simulink model "nuclearReactor"  (R2014b)
settings: Solver=ode1  StartTime=0.0  StopTime=100  FixedStep=0.0001  MaxStep=0.0001  RelTol=1e-3
(part 2 of 4)

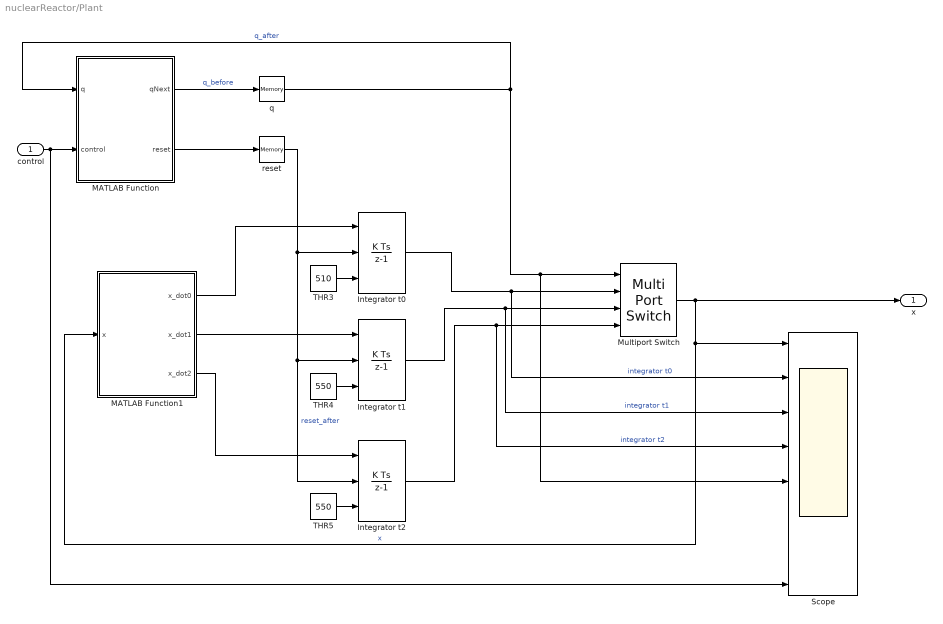
== system nuclearReactor/Plant ==
  control : Inport
  Integrator t0 : DiscreteIntegrator  ExternalReset=either  InitialConditionSource=external  InitialCondition=510  InitialConditionSetting=State (most efficient)  SampleTime=-1
  Integrator t1 : DiscreteIntegrator  ExternalReset=either  InitialConditionSource=external  InitialCondition=510  InitialConditionSetting=State (most efficient)  SampleTime=-1
  Integrator t2 : DiscreteIntegrator  ExternalReset=either  InitialConditionSource=external  InitialCondition=510  InitialConditionSetting=State (most efficient)  SampleTime=-1
  MATLAB Function : MATLAB Function  Priority=1  TreatAsAtomicUnit=on
  MATLAB Function1 : MATLAB Function  Priority=1  TreatAsAtomicUnit=on
  Multiport Switch : MultiPortSwitch  DataPortOrder=Zero-based contiguous
  Scope : Scope  NumInputPorts=8
      settings: TickLabels=on  ShowLegends=on  YMin=0~0~0~10~1~1~0~-1  YMax=40~20~20~30~3~3~1~1
  THR3 : Constant  Value=510
  THR4 : Constant  Value=550
  THR5 : Constant  Value=550
  q : Memory  LinearizeMemory=on
  reset : Memory  LinearizeMemory=on
  x : Outport
  wires:
  Multiport Switch/1 -> Scope/1, MATLAB Function1/1(x), x/1  "x"
  MATLAB Function1/1(x_dot0) -> Integrator t0/1
  THR3/1 -> Integrator t0/3
  THR4/1 -> Integrator t1/3
  THR5/1 -> Integrator t2/3
  Integrator t0/1 -> Scope/2, Multiport Switch/2  "integrator t0"
  Integrator t1/1 -> Scope/3, Multiport Switch/3  "integrator t1"
  Integrator t2/1 -> Scope/4, Multiport Switch/4  "integrator t2"
  MATLAB Function1/2(x_dot1) -> Integrator t1/1
  MATLAB Function1/3(x_dot2) -> Integrator t2/1
  MATLAB Function/1(qNext) -> q/1  "q_before"
  q/1 -> MATLAB Function/1(q), Scope/5, Multiport Switch/1  "q_after"
  control/1 -> Scope/8, MATLAB Function/2(control)
  MATLAB Function/2(reset) -> reset/1
  reset/1 -> Integrator t0/2, Integrator t1/2, Integrator t2/2  "reset_after"

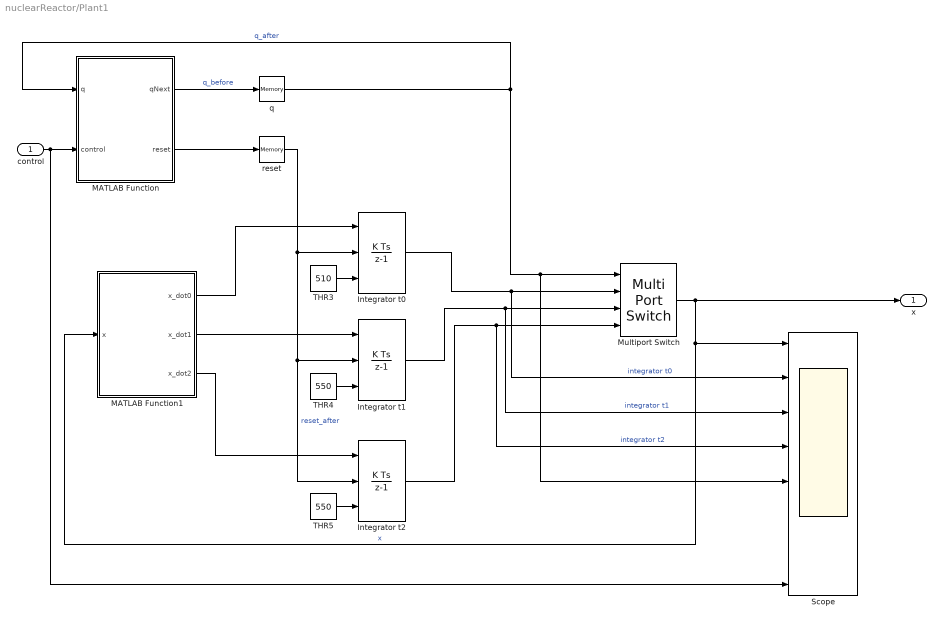
== system nuclearReactor/Plant1 ==
  control : Inport
  Integrator t0 : DiscreteIntegrator  ExternalReset=either  InitialConditionSource=external  InitialCondition=510  InitialConditionSetting=State (most efficient)  SampleTime=-1
  Integrator t1 : DiscreteIntegrator  ExternalReset=either  InitialConditionSource=external  InitialCondition=510  InitialConditionSetting=State (most efficient)  SampleTime=-1
  Integrator t2 : DiscreteIntegrator  ExternalReset=either  InitialConditionSource=external  InitialCondition=510  InitialConditionSetting=State (most efficient)  SampleTime=-1
  MATLAB Function : MATLAB Function  Priority=1  TreatAsAtomicUnit=on
  MATLAB Function1 : MATLAB Function  Priority=1  TreatAsAtomicUnit=on
  Multiport Switch : MultiPortSwitch  DataPortOrder=Zero-based contiguous
  Scope : Scope  NumInputPorts=8
      settings: TickLabels=on  ShowLegends=on  YMin=0~0~0~10~1~1~0~-1  YMax=40~20~20~30~3~3~1~1
  THR3 : Constant  Value=510
  THR4 : Constant  Value=550
  THR5 : Constant  Value=550
  q : Memory  LinearizeMemory=on
  reset : Memory  LinearizeMemory=on
  x : Outport
  wires:
  Multiport Switch/1 -> Scope/1, MATLAB Function1/1(x), x/1  "x"
  MATLAB Function1/1(x_dot0) -> Integrator t0/1
  THR3/1 -> Integrator t0/3
  THR4/1 -> Integrator t1/3
  THR5/1 -> Integrator t2/3
  Integrator t0/1 -> Scope/2, Multiport Switch/2  "integrator t0"
  Integrator t1/1 -> Scope/3, Multiport Switch/3  "integrator t1"
  Integrator t2/1 -> Scope/4, Multiport Switch/4  "integrator t2"
  MATLAB Function1/2(x_dot1) -> Integrator t1/1
  MATLAB Function1/3(x_dot2) -> Integrator t2/1
  MATLAB Function/1(qNext) -> q/1  "q_before"
  q/1 -> MATLAB Function/1(q), Scope/5, Multiport Switch/1  "q_after"
  control/1 -> Scope/8, MATLAB Function/2(control)
  MATLAB Function/2(reset) -> reset/1
  reset/1 -> Integrator t0/2, Integrator t1/2, Integrator t2/2  "reset_after"

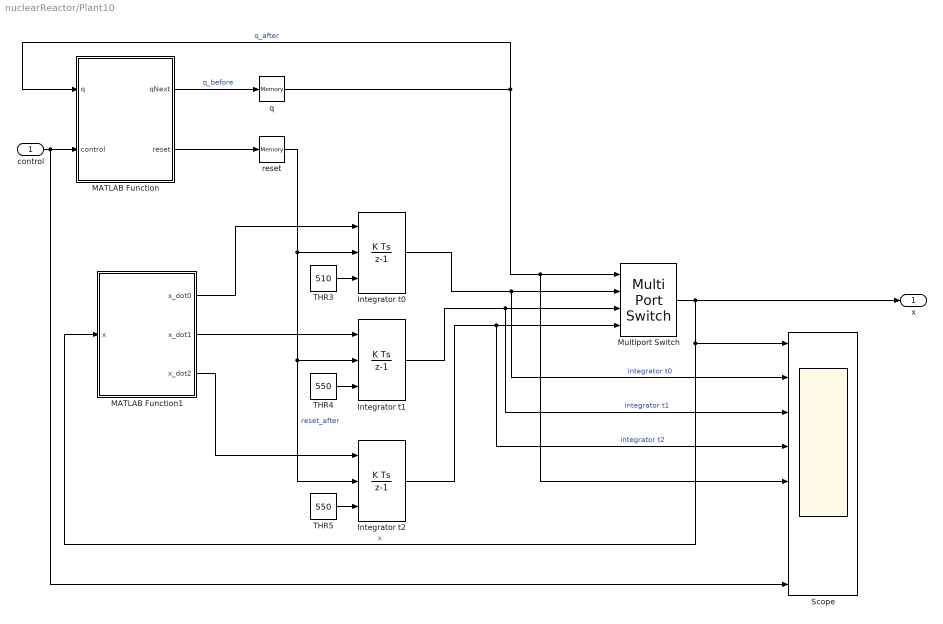
== system nuclearReactor/Plant10 ==
  control : Inport
  Integrator t0 : DiscreteIntegrator  ExternalReset=either  InitialConditionSource=external  InitialCondition=510  InitialConditionSetting=State (most efficient)  SampleTime=-1
  Integrator t1 : DiscreteIntegrator  ExternalReset=either  InitialConditionSource=external  InitialCondition=510  InitialConditionSetting=State (most efficient)  SampleTime=-1
  Integrator t2 : DiscreteIntegrator  ExternalReset=either  InitialConditionSource=external  InitialCondition=510  InitialConditionSetting=State (most efficient)  SampleTime=-1
  MATLAB Function : MATLAB Function  Priority=1  TreatAsAtomicUnit=on
  MATLAB Function1 : MATLAB Function  Priority=1  TreatAsAtomicUnit=on
  Multiport Switch : MultiPortSwitch  DataPortOrder=Zero-based contiguous
  Scope : Scope  NumInputPorts=8
      settings: TickLabels=on  ShowLegends=on  YMin=0~0~0~10~1~1~0~-1  YMax=40~20~20~30~3~3~1~1
  THR3 : Constant  Value=510
  THR4 : Constant  Value=550
  THR5 : Constant  Value=550
  q : Memory  LinearizeMemory=on
  reset : Memory  LinearizeMemory=on
  x : Outport
  wires:
  Multiport Switch/1 -> Scope/1, MATLAB Function1/1(x), x/1  "x"
  MATLAB Function1/1(x_dot0) -> Integrator t0/1
  THR3/1 -> Integrator t0/3
  THR4/1 -> Integrator t1/3
  THR5/1 -> Integrator t2/3
  Integrator t0/1 -> Scope/2, Multiport Switch/2  "integrator t0"
  Integrator t1/1 -> Scope/3, Multiport Switch/3  "integrator t1"
  Integrator t2/1 -> Scope/4, Multiport Switch/4  "integrator t2"
  MATLAB Function1/2(x_dot1) -> Integrator t1/1
  MATLAB Function1/3(x_dot2) -> Integrator t2/1
  MATLAB Function/1(qNext) -> q/1  "q_before"
  q/1 -> MATLAB Function/1(q), Scope/5, Multiport Switch/1  "q_after"
  control/1 -> Scope/8, MATLAB Function/2(control)
  MATLAB Function/2(reset) -> reset/1
  reset/1 -> Integrator t0/2, Integrator t1/2, Integrator t2/2  "reset_after"

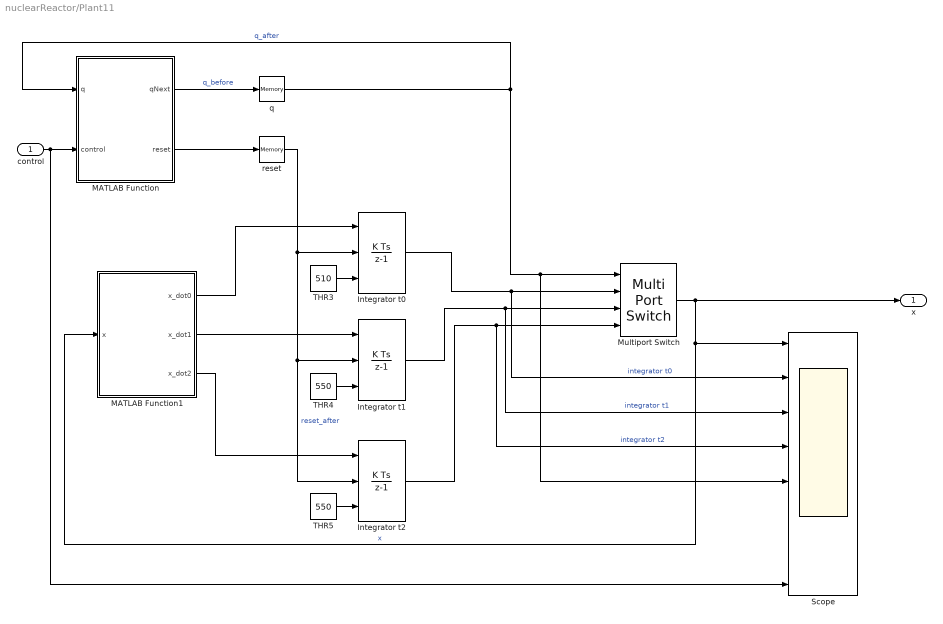
== system nuclearReactor/Plant11 ==
  control : Inport
  Integrator t0 : DiscreteIntegrator  ExternalReset=either  InitialConditionSource=external  InitialCondition=510  InitialConditionSetting=State (most efficient)  SampleTime=-1
  Integrator t1 : DiscreteIntegrator  ExternalReset=either  InitialConditionSource=external  InitialCondition=510  InitialConditionSetting=State (most efficient)  SampleTime=-1
  Integrator t2 : DiscreteIntegrator  ExternalReset=either  InitialConditionSource=external  InitialCondition=510  InitialConditionSetting=State (most efficient)  SampleTime=-1
  MATLAB Function : MATLAB Function  Priority=1  TreatAsAtomicUnit=on
  MATLAB Function1 : MATLAB Function  Priority=1  TreatAsAtomicUnit=on
  Multiport Switch : MultiPortSwitch  DataPortOrder=Zero-based contiguous
  Scope : Scope  NumInputPorts=8
      settings: TickLabels=on  ShowLegends=on  YMin=0~0~0~10~1~1~0~-1  YMax=40~20~20~30~3~3~1~1
  THR3 : Constant  Value=510
  THR4 : Constant  Value=550
  THR5 : Constant  Value=550
  q : Memory  LinearizeMemory=on
  reset : Memory  LinearizeMemory=on
  x : Outport
  wires:
  Multiport Switch/1 -> Scope/1, MATLAB Function1/1(x), x/1  "x"
  MATLAB Function1/1(x_dot0) -> Integrator t0/1
  THR3/1 -> Integrator t0/3
  THR4/1 -> Integrator t1/3
  THR5/1 -> Integrator t2/3
  Integrator t0/1 -> Scope/2, Multiport Switch/2  "integrator t0"
  Integrator t1/1 -> Scope/3, Multiport Switch/3  "integrator t1"
  Integrator t2/1 -> Scope/4, Multiport Switch/4  "integrator t2"
  MATLAB Function1/2(x_dot1) -> Integrator t1/1
  MATLAB Function1/3(x_dot2) -> Integrator t2/1
  MATLAB Function/1(qNext) -> q/1  "q_before"
  q/1 -> MATLAB Function/1(q), Scope/5, Multiport Switch/1  "q_after"
  control/1 -> Scope/8, MATLAB Function/2(control)
  MATLAB Function/2(reset) -> reset/1
  reset/1 -> Integrator t0/2, Integrator t1/2, Integrator t2/2  "reset_after"

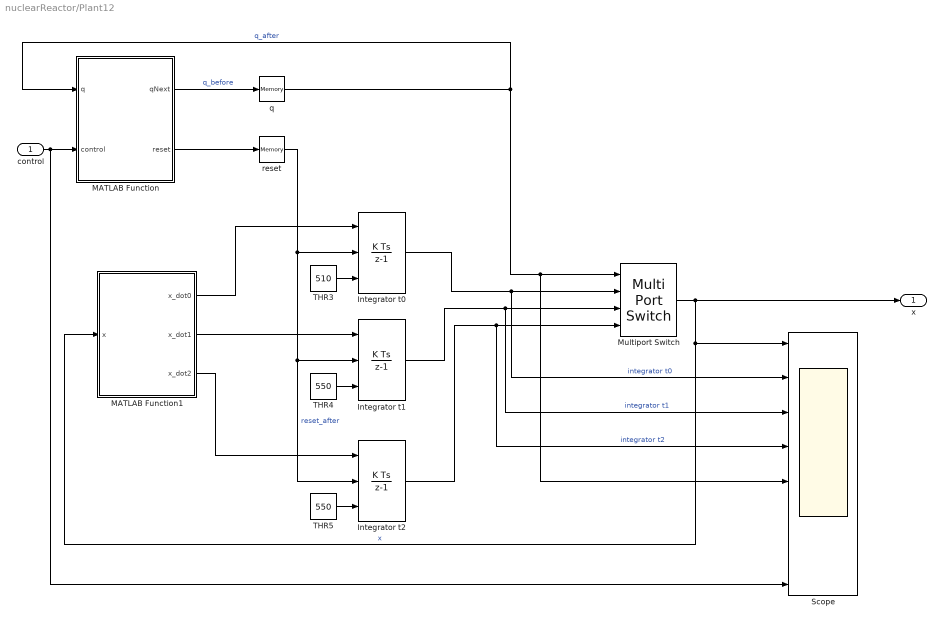
== system nuclearReactor/Plant12 ==
  control : Inport
  Integrator t0 : DiscreteIntegrator  ExternalReset=either  InitialConditionSource=external  InitialCondition=510  InitialConditionSetting=State (most efficient)  SampleTime=-1
  Integrator t1 : DiscreteIntegrator  ExternalReset=either  InitialConditionSource=external  InitialCondition=510  InitialConditionSetting=State (most efficient)  SampleTime=-1
  Integrator t2 : DiscreteIntegrator  ExternalReset=either  InitialConditionSource=external  InitialCondition=510  InitialConditionSetting=State (most efficient)  SampleTime=-1
  MATLAB Function : MATLAB Function  Priority=1  TreatAsAtomicUnit=on
  MATLAB Function1 : MATLAB Function  Priority=1  TreatAsAtomicUnit=on
  Multiport Switch : MultiPortSwitch  DataPortOrder=Zero-based contiguous
  Scope : Scope  NumInputPorts=8
      settings: TickLabels=on  ShowLegends=on  YMin=0~0~0~10~1~1~0~-1  YMax=40~20~20~30~3~3~1~1
  THR3 : Constant  Value=510
  THR4 : Constant  Value=550
  THR5 : Constant  Value=550
  q : Memory  LinearizeMemory=on
  reset : Memory  LinearizeMemory=on
  x : Outport
  wires:
  Multiport Switch/1 -> Scope/1, MATLAB Function1/1(x), x/1  "x"
  MATLAB Function1/1(x_dot0) -> Integrator t0/1
  THR3/1 -> Integrator t0/3
  THR4/1 -> Integrator t1/3
  THR5/1 -> Integrator t2/3
  Integrator t0/1 -> Scope/2, Multiport Switch/2  "integrator t0"
  Integrator t1/1 -> Scope/3, Multiport Switch/3  "integrator t1"
  Integrator t2/1 -> Scope/4, Multiport Switch/4  "integrator t2"
  MATLAB Function1/2(x_dot1) -> Integrator t1/1
  MATLAB Function1/3(x_dot2) -> Integrator t2/1
  MATLAB Function/1(qNext) -> q/1  "q_before"
  q/1 -> MATLAB Function/1(q), Scope/5, Multiport Switch/1  "q_after"
  control/1 -> Scope/8, MATLAB Function/2(control)
  MATLAB Function/2(reset) -> reset/1
  reset/1 -> Integrator t0/2, Integrator t1/2, Integrator t2/2  "reset_after"

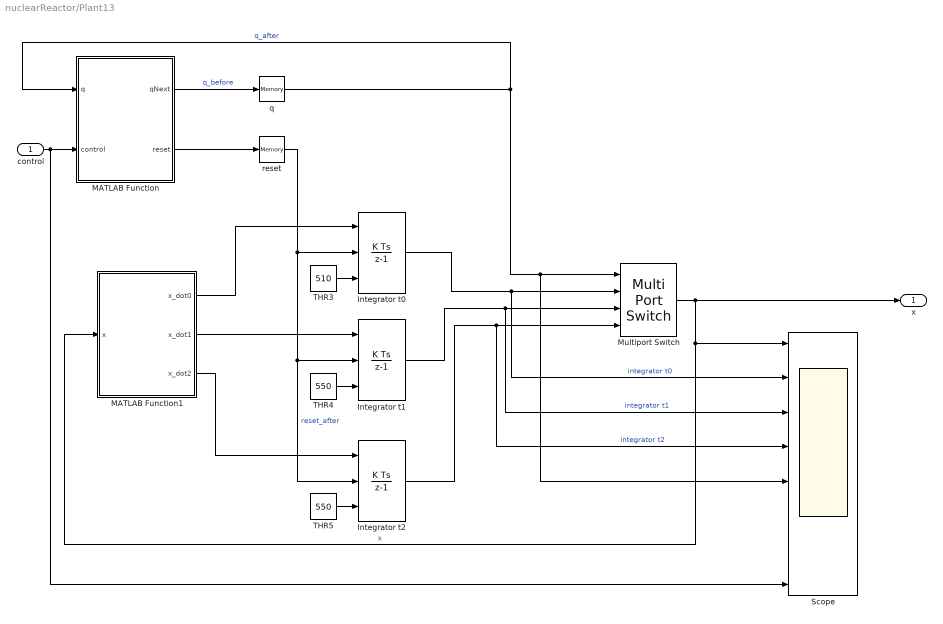
== system nuclearReactor/Plant13 ==
  control : Inport
  Integrator t0 : DiscreteIntegrator  ExternalReset=either  InitialConditionSource=external  InitialCondition=510  InitialConditionSetting=State (most efficient)  SampleTime=-1
  Integrator t1 : DiscreteIntegrator  ExternalReset=either  InitialConditionSource=external  InitialCondition=510  InitialConditionSetting=State (most efficient)  SampleTime=-1
  Integrator t2 : DiscreteIntegrator  ExternalReset=either  InitialConditionSource=external  InitialCondition=510  InitialConditionSetting=State (most efficient)  SampleTime=-1
  MATLAB Function : MATLAB Function  Priority=1  TreatAsAtomicUnit=on
  MATLAB Function1 : MATLAB Function  Priority=1  TreatAsAtomicUnit=on
  Multiport Switch : MultiPortSwitch  DataPortOrder=Zero-based contiguous
  Scope : Scope  NumInputPorts=8
      settings: TickLabels=on  ShowLegends=on  YMin=0~0~0~10~1~1~0~-1  YMax=40~20~20~30~3~3~1~1
  THR3 : Constant  Value=510
  THR4 : Constant  Value=550
  THR5 : Constant  Value=550
  q : Memory  LinearizeMemory=on
  reset : Memory  LinearizeMemory=on
  x : Outport
  wires:
  Multiport Switch/1 -> Scope/1, MATLAB Function1/1(x), x/1  "x"
  MATLAB Function1/1(x_dot0) -> Integrator t0/1
  THR3/1 -> Integrator t0/3
  THR4/1 -> Integrator t1/3
  THR5/1 -> Integrator t2/3
  Integrator t0/1 -> Scope/2, Multiport Switch/2  "integrator t0"
  Integrator t1/1 -> Scope/3, Multiport Switch/3  "integrator t1"
  Integrator t2/1 -> Scope/4, Multiport Switch/4  "integrator t2"
  MATLAB Function1/2(x_dot1) -> Integrator t1/1
  MATLAB Function1/3(x_dot2) -> Integrator t2/1
  MATLAB Function/1(qNext) -> q/1  "q_before"
  q/1 -> MATLAB Function/1(q), Scope/5, Multiport Switch/1  "q_after"
  control/1 -> Scope/8, MATLAB Function/2(control)
  MATLAB Function/2(reset) -> reset/1
  reset/1 -> Integrator t0/2, Integrator t1/2, Integrator t2/2  "reset_after"

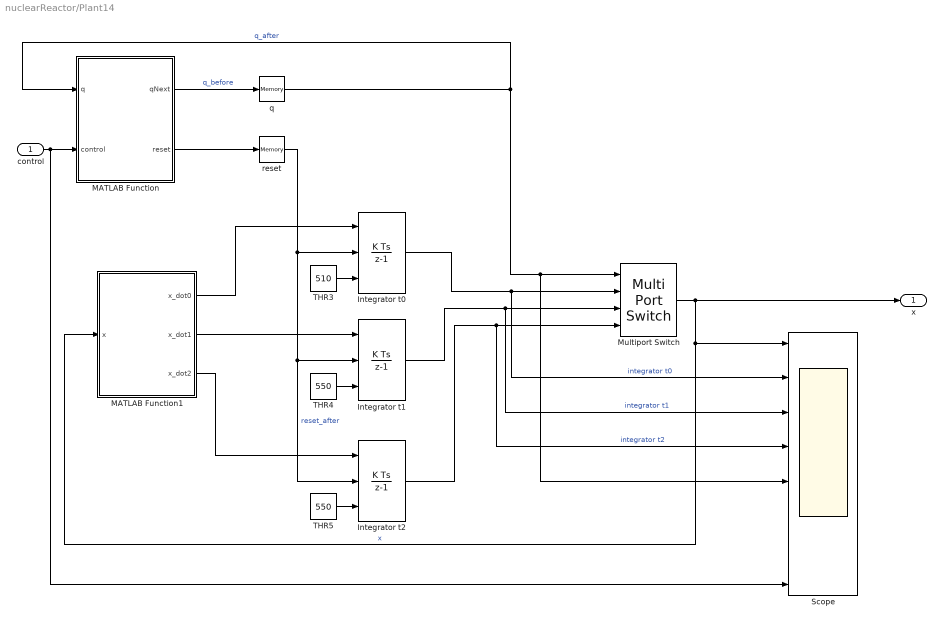
== system nuclearReactor/Plant14 ==
  control : Inport
  Integrator t0 : DiscreteIntegrator  ExternalReset=either  InitialConditionSource=external  InitialCondition=510  InitialConditionSetting=State (most efficient)  SampleTime=-1
  Integrator t1 : DiscreteIntegrator  ExternalReset=either  InitialConditionSource=external  InitialCondition=510  InitialConditionSetting=State (most efficient)  SampleTime=-1
  Integrator t2 : DiscreteIntegrator  ExternalReset=either  InitialConditionSource=external  InitialCondition=510  InitialConditionSetting=State (most efficient)  SampleTime=-1
  MATLAB Function : MATLAB Function  Priority=1  TreatAsAtomicUnit=on
  MATLAB Function1 : MATLAB Function  Priority=1  TreatAsAtomicUnit=on
  Multiport Switch : MultiPortSwitch  DataPortOrder=Zero-based contiguous
  Scope : Scope  NumInputPorts=8
      settings: TickLabels=on  ShowLegends=on  YMin=0~0~0~10~1~1~0~-1  YMax=40~20~20~30~3~3~1~1
  THR3 : Constant  Value=510
  THR4 : Constant  Value=550
  THR5 : Constant  Value=550
  q : Memory  LinearizeMemory=on
  reset : Memory  LinearizeMemory=on
  x : Outport
  wires:
  Multiport Switch/1 -> Scope/1, MATLAB Function1/1(x), x/1  "x"
  MATLAB Function1/1(x_dot0) -> Integrator t0/1
  THR3/1 -> Integrator t0/3
  THR4/1 -> Integrator t1/3
  THR5/1 -> Integrator t2/3
  Integrator t0/1 -> Scope/2, Multiport Switch/2  "integrator t0"
  Integrator t1/1 -> Scope/3, Multiport Switch/3  "integrator t1"
  Integrator t2/1 -> Scope/4, Multiport Switch/4  "integrator t2"
  MATLAB Function1/2(x_dot1) -> Integrator t1/1
  MATLAB Function1/3(x_dot2) -> Integrator t2/1
  MATLAB Function/1(qNext) -> q/1  "q_before"
  q/1 -> MATLAB Function/1(q), Scope/5, Multiport Switch/1  "q_after"
  control/1 -> Scope/8, MATLAB Function/2(control)
  MATLAB Function/2(reset) -> reset/1
  reset/1 -> Integrator t0/2, Integrator t1/2, Integrator t2/2  "reset_after"

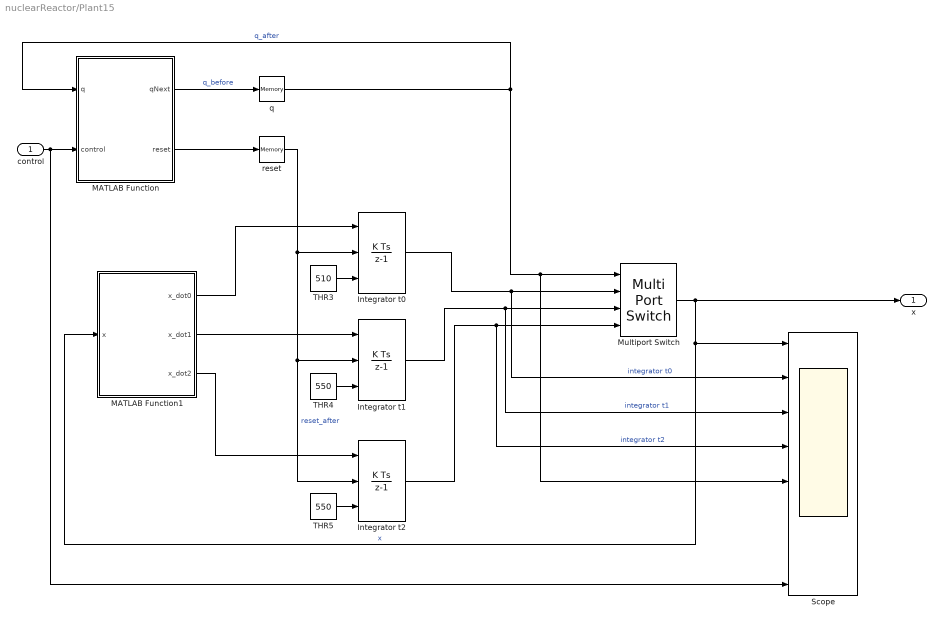
== system nuclearReactor/Plant15 ==
  control : Inport
  Integrator t0 : DiscreteIntegrator  ExternalReset=either  InitialConditionSource=external  InitialCondition=510  InitialConditionSetting=State (most efficient)  SampleTime=-1
  Integrator t1 : DiscreteIntegrator  ExternalReset=either  InitialConditionSource=external  InitialCondition=510  InitialConditionSetting=State (most efficient)  SampleTime=-1
  Integrator t2 : DiscreteIntegrator  ExternalReset=either  InitialConditionSource=external  InitialCondition=510  InitialConditionSetting=State (most efficient)  SampleTime=-1
  MATLAB Function : MATLAB Function  Priority=1  TreatAsAtomicUnit=on
  MATLAB Function1 : MATLAB Function  Priority=1  TreatAsAtomicUnit=on
  Multiport Switch : MultiPortSwitch  DataPortOrder=Zero-based contiguous
  Scope : Scope  NumInputPorts=8
      settings: TickLabels=on  ShowLegends=on  YMin=0~0~0~10~1~1~0~-1  YMax=40~20~20~30~3~3~1~1
  THR3 : Constant  Value=510
  THR4 : Constant  Value=550
  THR5 : Constant  Value=550
  q : Memory  LinearizeMemory=on
  reset : Memory  LinearizeMemory=on
  x : Outport
  wires:
  Multiport Switch/1 -> Scope/1, MATLAB Function1/1(x), x/1  "x"
  MATLAB Function1/1(x_dot0) -> Integrator t0/1
  THR3/1 -> Integrator t0/3
  THR4/1 -> Integrator t1/3
  THR5/1 -> Integrator t2/3
  Integrator t0/1 -> Scope/2, Multiport Switch/2  "integrator t0"
  Integrator t1/1 -> Scope/3, Multiport Switch/3  "integrator t1"
  Integrator t2/1 -> Scope/4, Multiport Switch/4  "integrator t2"
  MATLAB Function1/2(x_dot1) -> Integrator t1/1
  MATLAB Function1/3(x_dot2) -> Integrator t2/1
  MATLAB Function/1(qNext) -> q/1  "q_before"
  q/1 -> MATLAB Function/1(q), Scope/5, Multiport Switch/1  "q_after"
  control/1 -> Scope/8, MATLAB Function/2(control)
  MATLAB Function/2(reset) -> reset/1
  reset/1 -> Integrator t0/2, Integrator t1/2, Integrator t2/2  "reset_after"

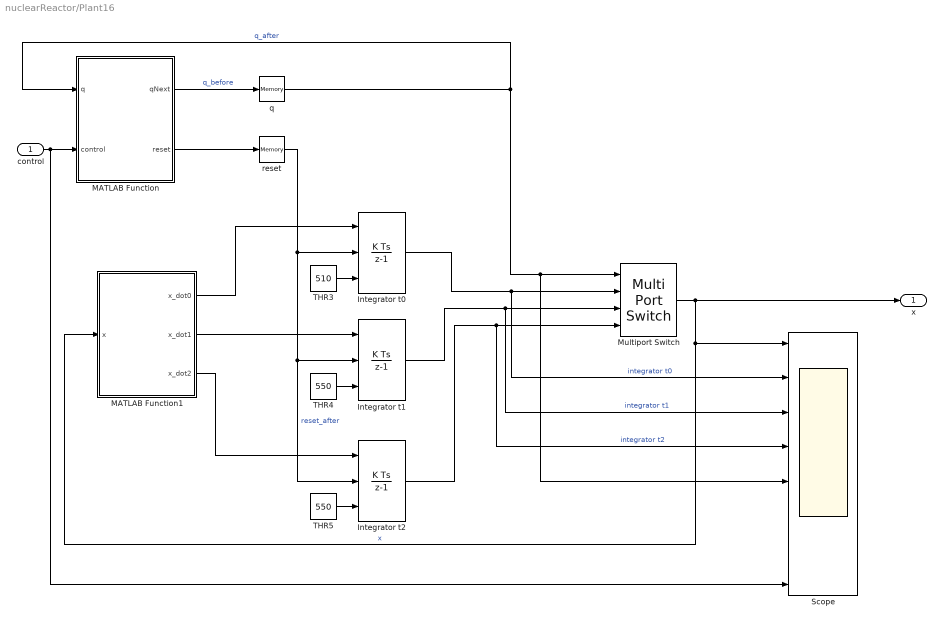
== system nuclearReactor/Plant16 ==
  control : Inport
  Integrator t0 : DiscreteIntegrator  ExternalReset=either  InitialConditionSource=external  InitialCondition=510  InitialConditionSetting=State (most efficient)  SampleTime=-1
  Integrator t1 : DiscreteIntegrator  ExternalReset=either  InitialConditionSource=external  InitialCondition=510  InitialConditionSetting=State (most efficient)  SampleTime=-1
  Integrator t2 : DiscreteIntegrator  ExternalReset=either  InitialConditionSource=external  InitialCondition=510  InitialConditionSetting=State (most efficient)  SampleTime=-1
  MATLAB Function : MATLAB Function  Priority=1  TreatAsAtomicUnit=on
  MATLAB Function1 : MATLAB Function  Priority=1  TreatAsAtomicUnit=on
  Multiport Switch : MultiPortSwitch  DataPortOrder=Zero-based contiguous
  Scope : Scope  NumInputPorts=8
      settings: TickLabels=on  ShowLegends=on  YMin=0~0~0~10~1~1~0~-1  YMax=40~20~20~30~3~3~1~1
  THR3 : Constant  Value=510
  THR4 : Constant  Value=550
  THR5 : Constant  Value=550
  q : Memory  LinearizeMemory=on
  reset : Memory  LinearizeMemory=on
  x : Outport
  wires:
  Multiport Switch/1 -> Scope/1, MATLAB Function1/1(x), x/1  "x"
  MATLAB Function1/1(x_dot0) -> Integrator t0/1
  THR3/1 -> Integrator t0/3
  THR4/1 -> Integrator t1/3
  THR5/1 -> Integrator t2/3
  Integrator t0/1 -> Scope/2, Multiport Switch/2  "integrator t0"
  Integrator t1/1 -> Scope/3, Multiport Switch/3  "integrator t1"
  Integrator t2/1 -> Scope/4, Multiport Switch/4  "integrator t2"
  MATLAB Function1/2(x_dot1) -> Integrator t1/1
  MATLAB Function1/3(x_dot2) -> Integrator t2/1
  MATLAB Function/1(qNext) -> q/1  "q_before"
  q/1 -> MATLAB Function/1(q), Scope/5, Multiport Switch/1  "q_after"
  control/1 -> Scope/8, MATLAB Function/2(control)
  MATLAB Function/2(reset) -> reset/1
  reset/1 -> Integrator t0/2, Integrator t1/2, Integrator t2/2  "reset_after"

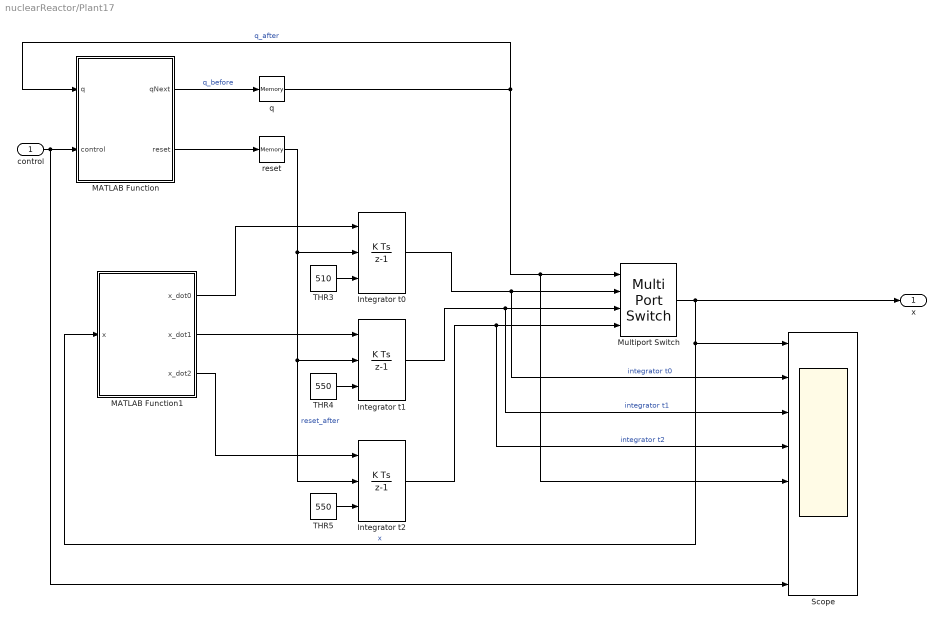
== system nuclearReactor/Plant17 ==
  control : Inport
  Integrator t0 : DiscreteIntegrator  ExternalReset=either  InitialConditionSource=external  InitialCondition=510  InitialConditionSetting=State (most efficient)  SampleTime=-1
  Integrator t1 : DiscreteIntegrator  ExternalReset=either  InitialConditionSource=external  InitialCondition=510  InitialConditionSetting=State (most efficient)  SampleTime=-1
  Integrator t2 : DiscreteIntegrator  ExternalReset=either  InitialConditionSource=external  InitialCondition=510  InitialConditionSetting=State (most efficient)  SampleTime=-1
  MATLAB Function : MATLAB Function  Priority=1  TreatAsAtomicUnit=on
  MATLAB Function1 : MATLAB Function  Priority=1  TreatAsAtomicUnit=on
  Multiport Switch : MultiPortSwitch  DataPortOrder=Zero-based contiguous
  Scope : Scope  NumInputPorts=8
      settings: TickLabels=on  ShowLegends=on  YMin=0~0~0~10~1~1~0~-1  YMax=40~20~20~30~3~3~1~1
  THR3 : Constant  Value=510
  THR4 : Constant  Value=550
  THR5 : Constant  Value=550
  q : Memory  LinearizeMemory=on
  reset : Memory  LinearizeMemory=on
  x : Outport
  wires:
  Multiport Switch/1 -> Scope/1, MATLAB Function1/1(x), x/1  "x"
  MATLAB Function1/1(x_dot0) -> Integrator t0/1
  THR3/1 -> Integrator t0/3
  THR4/1 -> Integrator t1/3
  THR5/1 -> Integrator t2/3
  Integrator t0/1 -> Scope/2, Multiport Switch/2  "integrator t0"
  Integrator t1/1 -> Scope/3, Multiport Switch/3  "integrator t1"
  Integrator t2/1 -> Scope/4, Multiport Switch/4  "integrator t2"
  MATLAB Function1/2(x_dot1) -> Integrator t1/1
  MATLAB Function1/3(x_dot2) -> Integrator t2/1
  MATLAB Function/1(qNext) -> q/1  "q_before"
  q/1 -> MATLAB Function/1(q), Scope/5, Multiport Switch/1  "q_after"
  control/1 -> Scope/8, MATLAB Function/2(control)
  MATLAB Function/2(reset) -> reset/1
  reset/1 -> Integrator t0/2, Integrator t1/2, Integrator t2/2  "reset_after"

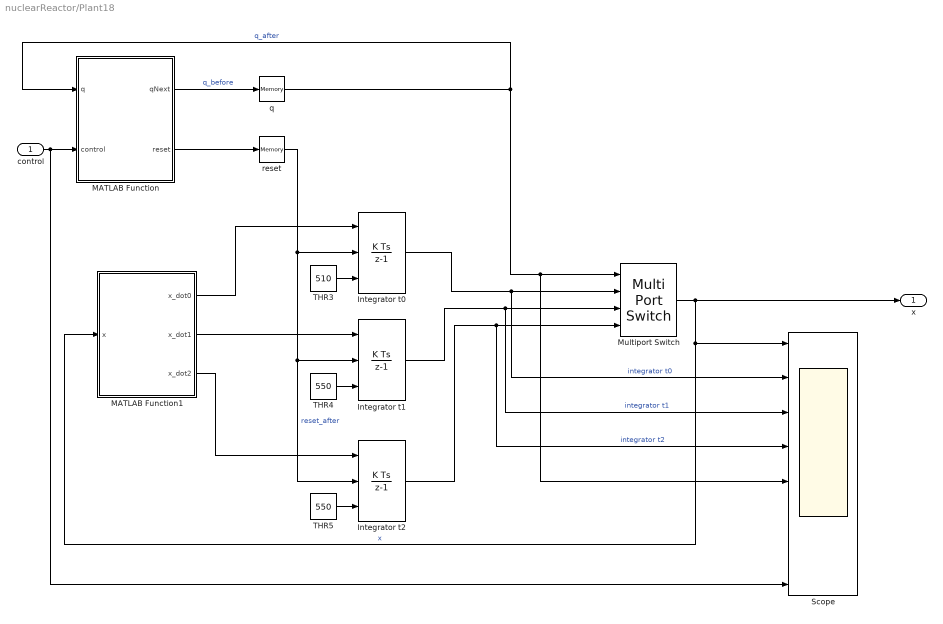
== system nuclearReactor/Plant18 ==
  control : Inport
  Integrator t0 : DiscreteIntegrator  ExternalReset=either  InitialConditionSource=external  InitialCondition=510  InitialConditionSetting=State (most efficient)  SampleTime=-1
  Integrator t1 : DiscreteIntegrator  ExternalReset=either  InitialConditionSource=external  InitialCondition=510  InitialConditionSetting=State (most efficient)  SampleTime=-1
  Integrator t2 : DiscreteIntegrator  ExternalReset=either  InitialConditionSource=external  InitialCondition=510  InitialConditionSetting=State (most efficient)  SampleTime=-1
  MATLAB Function : MATLAB Function  Priority=1  TreatAsAtomicUnit=on
  MATLAB Function1 : MATLAB Function  Priority=1  TreatAsAtomicUnit=on
  Multiport Switch : MultiPortSwitch  DataPortOrder=Zero-based contiguous
  Scope : Scope  NumInputPorts=8
      settings: TickLabels=on  ShowLegends=on  YMin=0~0~0~10~1~1~0~-1  YMax=40~20~20~30~3~3~1~1
  THR3 : Constant  Value=510
  THR4 : Constant  Value=550
  THR5 : Constant  Value=550
  q : Memory  LinearizeMemory=on
  reset : Memory  LinearizeMemory=on
  x : Outport
  wires:
  Multiport Switch/1 -> Scope/1, MATLAB Function1/1(x), x/1  "x"
  MATLAB Function1/1(x_dot0) -> Integrator t0/1
  THR3/1 -> Integrator t0/3
  THR4/1 -> Integrator t1/3
  THR5/1 -> Integrator t2/3
  Integrator t0/1 -> Scope/2, Multiport Switch/2  "integrator t0"
  Integrator t1/1 -> Scope/3, Multiport Switch/3  "integrator t1"
  Integrator t2/1 -> Scope/4, Multiport Switch/4  "integrator t2"
  MATLAB Function1/2(x_dot1) -> Integrator t1/1
  MATLAB Function1/3(x_dot2) -> Integrator t2/1
  MATLAB Function/1(qNext) -> q/1  "q_before"
  q/1 -> MATLAB Function/1(q), Scope/5, Multiport Switch/1  "q_after"
  control/1 -> Scope/8, MATLAB Function/2(control)
  MATLAB Function/2(reset) -> reset/1
  reset/1 -> Integrator t0/2, Integrator t1/2, Integrator t2/2  "reset_after"

== system nuclearReactor/Plant19 ==
  control : Inport
  Integrator t0 : DiscreteIntegrator  ExternalReset=either  InitialConditionSource=external  InitialCondition=510  InitialConditionSetting=State (most efficient)  SampleTime=-1
  Integrator t1 : DiscreteIntegrator  ExternalReset=either  InitialConditionSource=external  InitialCondition=510  InitialConditionSetting=State (most efficient)  SampleTime=-1
  Integrator t2 : DiscreteIntegrator  ExternalReset=either  InitialConditionSource=external  InitialCondition=510  InitialConditionSetting=State (most efficient)  SampleTime=-1
  MATLAB Function : MATLAB Function  Priority=1  TreatAsAtomicUnit=on
  MATLAB Function1 : MATLAB Function  Priority=1  TreatAsAtomicUnit=on
  Multiport Switch : MultiPortSwitch  DataPortOrder=Zero-based contiguous
  Scope : Scope  NumInputPorts=8
      settings: TickLabels=on  ShowLegends=on  YMin=0~0~0~10~1~1~0~-1  YMax=40~20~20~30~3~3~1~1
  THR3 : Constant  Value=510
  THR4 : Constant  Value=550
  THR5 : Constant  Value=550
  q : Memory  LinearizeMemory=on
  reset : Memory  LinearizeMemory=on
  x : Outport
  wires:
  Multiport Switch/1 -> Scope/1, MATLAB Function1/1(x), x/1  "x"
  MATLAB Function1/1(x_dot0) -> Integrator t0/1
  THR3/1 -> Integrator t0/3
  THR4/1 -> Integrator t1/3
  THR5/1 -> Integrator t2/3
  Integrator t0/1 -> Scope/2, Multiport Switch/2  "integrator t0"
  Integrator t1/1 -> Scope/3, Multiport Switch/3  "integrator t1"
  Integrator t2/1 -> Scope/4, Multiport Switch/4  "integrator t2"
  MATLAB Function1/2(x_dot1) -> Integrator t1/1
  MATLAB Function1/3(x_dot2) -> Integrator t2/1
  MATLAB Function/1(qNext) -> q/1  "q_before"
  q/1 -> MATLAB Function/1(q), Scope/5, Multiport Switch/1  "q_after"
  control/1 -> Scope/8, MATLAB Function/2(control)
  MATLAB Function/2(reset) -> reset/1
  reset/1 -> Integrator t0/2, Integrator t1/2, Integrator t2/2  "reset_after"

== system nuclearReactor/Plant2 ==
  control : Inport
  Integrator t0 : DiscreteIntegrator  ExternalReset=either  InitialConditionSource=external  InitialCondition=510  InitialConditionSetting=State (most efficient)  SampleTime=-1
  Integrator t1 : DiscreteIntegrator  ExternalReset=either  InitialConditionSource=external  InitialCondition=510  InitialConditionSetting=State (most efficient)  SampleTime=-1
  Integrator t2 : DiscreteIntegrator  ExternalReset=either  InitialConditionSource=external  InitialCondition=510  InitialConditionSetting=State (most efficient)  SampleTime=-1
  MATLAB Function : MATLAB Function  Priority=1  TreatAsAtomicUnit=on
  MATLAB Function1 : MATLAB Function  Priority=1  TreatAsAtomicUnit=on
  Multiport Switch : MultiPortSwitch  DataPortOrder=Zero-based contiguous
  Scope : Scope  NumInputPorts=8
      settings: TickLabels=on  ShowLegends=on  YMin=0~0~0~10~1~1~0~-1  YMax=40~20~20~30~3~3~1~1
  THR3 : Constant  Value=510
  THR4 : Constant  Value=550
  THR5 : Constant  Value=550
  q : Memory  LinearizeMemory=on
  reset : Memory  LinearizeMemory=on
  x : Outport
  wires:
  Multiport Switch/1 -> Scope/1, MATLAB Function1/1(x), x/1  "x"
  MATLAB Function1/1(x_dot0) -> Integrator t0/1
  THR3/1 -> Integrator t0/3
  THR4/1 -> Integrator t1/3
  THR5/1 -> Integrator t2/3
  Integrator t0/1 -> Scope/2, Multiport Switch/2  "integrator t0"
  Integrator t1/1 -> Scope/3, Multiport Switch/3  "integrator t1"
  Integrator t2/1 -> Scope/4, Multiport Switch/4  "integrator t2"
  MATLAB Function1/2(x_dot1) -> Integrator t1/1
  MATLAB Function1/3(x_dot2) -> Integrator t2/1
  MATLAB Function/1(qNext) -> q/1  "q_before"
  q/1 -> MATLAB Function/1(q), Scope/5, Multiport Switch/1  "q_after"
  control/1 -> Scope/8, MATLAB Function/2(control)
  MATLAB Function/2(reset) -> reset/1
  reset/1 -> Integrator t0/2, Integrator t1/2, Integrator t2/2  "reset_after"

== system nuclearReactor/Plant20 ==
  control : Inport
  Integrator t0 : DiscreteIntegrator  ExternalReset=either  InitialConditionSource=external  InitialCondition=510  InitialConditionSetting=State (most efficient)  SampleTime=-1
  Integrator t1 : DiscreteIntegrator  ExternalReset=either  InitialConditionSource=external  InitialCondition=510  InitialConditionSetting=State (most efficient)  SampleTime=-1
  Integrator t2 : DiscreteIntegrator  ExternalReset=either  InitialConditionSource=external  InitialCondition=510  InitialConditionSetting=State (most efficient)  SampleTime=-1
  MATLAB Function : MATLAB Function  Priority=1  TreatAsAtomicUnit=on
  MATLAB Function1 : MATLAB Function  Priority=1  TreatAsAtomicUnit=on
  Multiport Switch : MultiPortSwitch  DataPortOrder=Zero-based contiguous
  Scope : Scope  NumInputPorts=8
      settings: TickLabels=on  ShowLegends=on  YMin=0~0~0~10~1~1~0~-1  YMax=40~20~20~30~3~3~1~1
  THR3 : Constant  Value=510
  THR4 : Constant  Value=550
  THR5 : Constant  Value=550
  q : Memory  LinearizeMemory=on
  reset : Memory  LinearizeMemory=on
  x : Outport
  wires:
  Multiport Switch/1 -> Scope/1, MATLAB Function1/1(x), x/1  "x"
  MATLAB Function1/1(x_dot0) -> Integrator t0/1
  THR3/1 -> Integrator t0/3
  THR4/1 -> Integrator t1/3
  THR5/1 -> Integrator t2/3
  Integrator t0/1 -> Scope/2, Multiport Switch/2  "integrator t0"
  Integrator t1/1 -> Scope/3, Multiport Switch/3  "integrator t1"
  Integrator t2/1 -> Scope/4, Multiport Switch/4  "integrator t2"
  MATLAB Function1/2(x_dot1) -> Integrator t1/1
  MATLAB Function1/3(x_dot2) -> Integrator t2/1
  MATLAB Function/1(qNext) -> q/1  "q_before"
  q/1 -> MATLAB Function/1(q), Scope/5, Multiport Switch/1  "q_after"
  control/1 -> Scope/8, MATLAB Function/2(control)
  MATLAB Function/2(reset) -> reset/1
  reset/1 -> Integrator t0/2, Integrator t1/2, Integrator t2/2  "reset_after"

== system nuclearReactor/Plant21 ==
  control : Inport
  Integrator t0 : DiscreteIntegrator  ExternalReset=either  InitialConditionSource=external  InitialCondition=510  InitialConditionSetting=State (most efficient)  SampleTime=-1
  Integrator t1 : DiscreteIntegrator  ExternalReset=either  InitialConditionSource=external  InitialCondition=510  InitialConditionSetting=State (most efficient)  SampleTime=-1
  Integrator t2 : DiscreteIntegrator  ExternalReset=either  InitialConditionSource=external  InitialCondition=510  InitialConditionSetting=State (most efficient)  SampleTime=-1
  MATLAB Function : MATLAB Function  Priority=1  TreatAsAtomicUnit=on
  MATLAB Function1 : MATLAB Function  Priority=1  TreatAsAtomicUnit=on
  Multiport Switch : MultiPortSwitch  DataPortOrder=Zero-based contiguous
  Scope : Scope  NumInputPorts=8
      settings: TickLabels=on  ShowLegends=on  YMin=0~0~0~10~1~1~0~-1  YMax=40~20~20~30~3~3~1~1
  THR3 : Constant  Value=510
  THR4 : Constant  Value=550
  THR5 : Constant  Value=550
  q : Memory  LinearizeMemory=on
  reset : Memory  LinearizeMemory=on
  x : Outport
  wires:
  Multiport Switch/1 -> Scope/1, MATLAB Function1/1(x), x/1  "x"
  MATLAB Function1/1(x_dot0) -> Integrator t0/1
  THR3/1 -> Integrator t0/3
  THR4/1 -> Integrator t1/3
  THR5/1 -> Integrator t2/3
  Integrator t0/1 -> Scope/2, Multiport Switch/2  "integrator t0"
  Integrator t1/1 -> Scope/3, Multiport Switch/3  "integrator t1"
  Integrator t2/1 -> Scope/4, Multiport Switch/4  "integrator t2"
  MATLAB Function1/2(x_dot1) -> Integrator t1/1
  MATLAB Function1/3(x_dot2) -> Integrator t2/1
  MATLAB Function/1(qNext) -> q/1  "q_before"
  q/1 -> MATLAB Function/1(q), Scope/5, Multiport Switch/1  "q_after"
  control/1 -> Scope/8, MATLAB Function/2(control)
  MATLAB Function/2(reset) -> reset/1
  reset/1 -> Integrator t0/2, Integrator t1/2, Integrator t2/2  "reset_after"

== system nuclearReactor/Plant22 ==
  control : Inport
  Integrator t0 : DiscreteIntegrator  ExternalReset=either  InitialConditionSource=external  InitialCondition=510  InitialConditionSetting=State (most efficient)  SampleTime=-1
  Integrator t1 : DiscreteIntegrator  ExternalReset=either  InitialConditionSource=external  InitialCondition=510  InitialConditionSetting=State (most efficient)  SampleTime=-1
  Integrator t2 : DiscreteIntegrator  ExternalReset=either  InitialConditionSource=external  InitialCondition=510  InitialConditionSetting=State (most efficient)  SampleTime=-1
  MATLAB Function : MATLAB Function  Priority=1  TreatAsAtomicUnit=on
  MATLAB Function1 : MATLAB Function  Priority=1  TreatAsAtomicUnit=on
  Multiport Switch : MultiPortSwitch  DataPortOrder=Zero-based contiguous
  Scope : Scope  NumInputPorts=8
      settings: TickLabels=on  ShowLegends=on  YMin=0~0~0~10~1~1~0~-1  YMax=40~20~20~30~3~3~1~1
  THR3 : Constant  Value=510
  THR4 : Constant  Value=550
  THR5 : Constant  Value=550
  q : Memory  LinearizeMemory=on
  reset : Memory  LinearizeMemory=on
  x : Outport
  wires:
  Multiport Switch/1 -> Scope/1, MATLAB Function1/1(x), x/1  "x"
  MATLAB Function1/1(x_dot0) -> Integrator t0/1
  THR3/1 -> Integrator t0/3
  THR4/1 -> Integrator t1/3
  THR5/1 -> Integrator t2/3
  Integrator t0/1 -> Scope/2, Multiport Switch/2  "integrator t0"
  Integrator t1/1 -> Scope/3, Multiport Switch/3  "integrator t1"
  Integrator t2/1 -> Scope/4, Multiport Switch/4  "integrator t2"
  MATLAB Function1/2(x_dot1) -> Integrator t1/1
  MATLAB Function1/3(x_dot2) -> Integrator t2/1
  MATLAB Function/1(qNext) -> q/1  "q_before"
  q/1 -> MATLAB Function/1(q), Scope/5, Multiport Switch/1  "q_after"
  control/1 -> Scope/8, MATLAB Function/2(control)
  MATLAB Function/2(reset) -> reset/1
  reset/1 -> Integrator t0/2, Integrator t1/2, Integrator t2/2  "reset_after"

== system nuclearReactor/Plant23 ==
  control : Inport
  Integrator t0 : DiscreteIntegrator  ExternalReset=either  InitialConditionSource=external  InitialCondition=510  InitialConditionSetting=State (most efficient)  SampleTime=-1
  Integrator t1 : DiscreteIntegrator  ExternalReset=either  InitialConditionSource=external  InitialCondition=510  InitialConditionSetting=State (most efficient)  SampleTime=-1
  Integrator t2 : DiscreteIntegrator  ExternalReset=either  InitialConditionSource=external  InitialCondition=510  InitialConditionSetting=State (most efficient)  SampleTime=-1
  MATLAB Function : MATLAB Function  Priority=1  TreatAsAtomicUnit=on
  MATLAB Function1 : MATLAB Function  Priority=1  TreatAsAtomicUnit=on
  Multiport Switch : MultiPortSwitch  DataPortOrder=Zero-based contiguous
  Scope : Scope  NumInputPorts=8
      settings: TickLabels=on  ShowLegends=on  YMin=0~0~0~10~1~1~0~-1  YMax=40~20~20~30~3~3~1~1
  THR3 : Constant  Value=510
  THR4 : Constant  Value=550
  THR5 : Constant  Value=550
  q : Memory  LinearizeMemory=on
  reset : Memory  LinearizeMemory=on
  x : Outport
  wires:
  Multiport Switch/1 -> Scope/1, MATLAB Function1/1(x), x/1  "x"
  MATLAB Function1/1(x_dot0) -> Integrator t0/1
  THR3/1 -> Integrator t0/3
  THR4/1 -> Integrator t1/3
  THR5/1 -> Integrator t2/3
  Integrator t0/1 -> Scope/2, Multiport Switch/2  "integrator t0"
  Integrator t1/1 -> Scope/3, Multiport Switch/3  "integrator t1"
  Integrator t2/1 -> Scope/4, Multiport Switch/4  "integrator t2"
  MATLAB Function1/2(x_dot1) -> Integrator t1/1
  MATLAB Function1/3(x_dot2) -> Integrator t2/1
  MATLAB Function/1(qNext) -> q/1  "q_before"
  q/1 -> MATLAB Function/1(q), Scope/5, Multiport Switch/1  "q_after"
  control/1 -> Scope/8, MATLAB Function/2(control)
  MATLAB Function/2(reset) -> reset/1
  reset/1 -> Integrator t0/2, Integrator t1/2, Integrator t2/2  "reset_after"

== system nuclearReactor/Plant24 ==
  control : Inport
  Integrator t0 : DiscreteIntegrator  ExternalReset=either  InitialConditionSource=external  InitialCondition=510  InitialConditionSetting=State (most efficient)  SampleTime=-1
  Integrator t1 : DiscreteIntegrator  ExternalReset=either  InitialConditionSource=external  InitialCondition=510  InitialConditionSetting=State (most efficient)  SampleTime=-1
  Integrator t2 : DiscreteIntegrator  ExternalReset=either  InitialConditionSource=external  InitialCondition=510  InitialConditionSetting=State (most efficient)  SampleTime=-1
  MATLAB Function : MATLAB Function  Priority=1  TreatAsAtomicUnit=on
  MATLAB Function1 : MATLAB Function  Priority=1  TreatAsAtomicUnit=on
  Multiport Switch : MultiPortSwitch  DataPortOrder=Zero-based contiguous
  Scope : Scope  NumInputPorts=8
      settings: TickLabels=on  ShowLegends=on  YMin=0~0~0~10~1~1~0~-1  YMax=40~20~20~30~3~3~1~1
  THR3 : Constant  Value=510
  THR4 : Constant  Value=550
  THR5 : Constant  Value=550
  q : Memory  LinearizeMemory=on
  reset : Memory  LinearizeMemory=on
  x : Outport
  wires:
  Multiport Switch/1 -> Scope/1, MATLAB Function1/1(x), x/1  "x"
  MATLAB Function1/1(x_dot0) -> Integrator t0/1
  THR3/1 -> Integrator t0/3
  THR4/1 -> Integrator t1/3
  THR5/1 -> Integrator t2/3
  Integrator t0/1 -> Scope/2, Multiport Switch/2  "integrator t0"
  Integrator t1/1 -> Scope/3, Multiport Switch/3  "integrator t1"
  Integrator t2/1 -> Scope/4, Multiport Switch/4  "integrator t2"
  MATLAB Function1/2(x_dot1) -> Integrator t1/1
  MATLAB Function1/3(x_dot2) -> Integrator t2/1
  MATLAB Function/1(qNext) -> q/1  "q_before"
  q/1 -> MATLAB Function/1(q), Scope/5, Multiport Switch/1  "q_after"
  control/1 -> Scope/8, MATLAB Function/2(control)
  MATLAB Function/2(reset) -> reset/1
  reset/1 -> Integrator t0/2, Integrator t1/2, Integrator t2/2  "reset_after"

== system nuclearReactor/Plant25 ==
  control : Inport
  Integrator t0 : DiscreteIntegrator  ExternalReset=either  InitialConditionSource=external  InitialCondition=510  InitialConditionSetting=State (most efficient)  SampleTime=-1
  Integrator t1 : DiscreteIntegrator  ExternalReset=either  InitialConditionSource=external  InitialCondition=510  InitialConditionSetting=State (most efficient)  SampleTime=-1
  Integrator t2 : DiscreteIntegrator  ExternalReset=either  InitialConditionSource=external  InitialCondition=510  InitialConditionSetting=State (most efficient)  SampleTime=-1
  MATLAB Function : MATLAB Function  Priority=1  TreatAsAtomicUnit=on
  MATLAB Function1 : MATLAB Function  Priority=1  TreatAsAtomicUnit=on
  Multiport Switch : MultiPortSwitch  DataPortOrder=Zero-based contiguous
  Scope : Scope  NumInputPorts=8
      settings: TickLabels=on  ShowLegends=on  YMin=0~0~0~10~1~1~0~-1  YMax=40~20~20~30~3~3~1~1
  THR3 : Constant  Value=510
  THR4 : Constant  Value=550
  THR5 : Constant  Value=550
  q : Memory  LinearizeMemory=on
  reset : Memory  LinearizeMemory=on
  x : Outport
  wires:
  Multiport Switch/1 -> Scope/1, MATLAB Function1/1(x), x/1  "x"
  MATLAB Function1/1(x_dot0) -> Integrator t0/1
  THR3/1 -> Integrator t0/3
  THR4/1 -> Integrator t1/3
  THR5/1 -> Integrator t2/3
  Integrator t0/1 -> Scope/2, Multiport Switch/2  "integrator t0"
  Integrator t1/1 -> Scope/3, Multiport Switch/3  "integrator t1"
  Integrator t2/1 -> Scope/4, Multiport Switch/4  "integrator t2"
  MATLAB Function1/2(x_dot1) -> Integrator t1/1
  MATLAB Function1/3(x_dot2) -> Integrator t2/1
  MATLAB Function/1(qNext) -> q/1  "q_before"
  q/1 -> MATLAB Function/1(q), Scope/5, Multiport Switch/1  "q_after"
  control/1 -> Scope/8, MATLAB Function/2(control)
  MATLAB Function/2(reset) -> reset/1
  reset/1 -> Integrator t0/2, Integrator t1/2, Integrator t2/2  "reset_after"

== system nuclearReactor/Plant26 ==
  control : Inport
  Integrator t0 : DiscreteIntegrator  ExternalReset=either  InitialConditionSource=external  InitialCondition=510  InitialConditionSetting=State (most efficient)  SampleTime=-1
  Integrator t1 : DiscreteIntegrator  ExternalReset=either  InitialConditionSource=external  InitialCondition=510  InitialConditionSetting=State (most efficient)  SampleTime=-1
  Integrator t2 : DiscreteIntegrator  ExternalReset=either  InitialConditionSource=external  InitialCondition=510  InitialConditionSetting=State (most efficient)  SampleTime=-1
  MATLAB Function : MATLAB Function  Priority=1  TreatAsAtomicUnit=on
  MATLAB Function1 : MATLAB Function  Priority=1  TreatAsAtomicUnit=on
  Multiport Switch : MultiPortSwitch  DataPortOrder=Zero-based contiguous
  Scope : Scope  NumInputPorts=8
      settings: TickLabels=on  ShowLegends=on  YMin=0~0~0~10~1~1~0~-1  YMax=40~20~20~30~3~3~1~1
  THR3 : Constant  Value=510
  THR4 : Constant  Value=550
  THR5 : Constant  Value=550
  q : Memory  LinearizeMemory=on
  reset : Memory  LinearizeMemory=on
  x : Outport
  wires:
  Multiport Switch/1 -> Scope/1, MATLAB Function1/1(x), x/1  "x"
  MATLAB Function1/1(x_dot0) -> Integrator t0/1
  THR3/1 -> Integrator t0/3
  THR4/1 -> Integrator t1/3
  THR5/1 -> Integrator t2/3
  Integrator t0/1 -> Scope/2, Multiport Switch/2  "integrator t0"
  Integrator t1/1 -> Scope/3, Multiport Switch/3  "integrator t1"
  Integrator t2/1 -> Scope/4, Multiport Switch/4  "integrator t2"
  MATLAB Function1/2(x_dot1) -> Integrator t1/1
  MATLAB Function1/3(x_dot2) -> Integrator t2/1
  MATLAB Function/1(qNext) -> q/1  "q_before"
  q/1 -> MATLAB Function/1(q), Scope/5, Multiport Switch/1  "q_after"
  control/1 -> Scope/8, MATLAB Function/2(control)
  MATLAB Function/2(reset) -> reset/1
  reset/1 -> Integrator t0/2, Integrator t1/2, Integrator t2/2  "reset_after"

== system nuclearReactor/Plant27 ==
  control : Inport
  Integrator t0 : DiscreteIntegrator  ExternalReset=either  InitialConditionSource=external  InitialCondition=510  InitialConditionSetting=State (most efficient)  SampleTime=-1
  Integrator t1 : DiscreteIntegrator  ExternalReset=either  InitialConditionSource=external  InitialCondition=510  InitialConditionSetting=State (most efficient)  SampleTime=-1
  Integrator t2 : DiscreteIntegrator  ExternalReset=either  InitialConditionSource=external  InitialCondition=510  InitialConditionSetting=State (most efficient)  SampleTime=-1
  MATLAB Function : MATLAB Function  Priority=1  TreatAsAtomicUnit=on
  MATLAB Function1 : MATLAB Function  Priority=1  TreatAsAtomicUnit=on
  Multiport Switch : MultiPortSwitch  DataPortOrder=Zero-based contiguous
  Scope : Scope  NumInputPorts=8
      settings: TickLabels=on  ShowLegends=on  YMin=0~0~0~10~1~1~0~-1  YMax=40~20~20~30~3~3~1~1
  THR3 : Constant  Value=510
  THR4 : Constant  Value=550
  THR5 : Constant  Value=550
  q : Memory  LinearizeMemory=on
  reset : Memory  LinearizeMemory=on
  x : Outport
  wires:
  Multiport Switch/1 -> Scope/1, MATLAB Function1/1(x), x/1  "x"
  MATLAB Function1/1(x_dot0) -> Integrator t0/1
  THR3/1 -> Integrator t0/3
  THR4/1 -> Integrator t1/3
  THR5/1 -> Integrator t2/3
  Integrator t0/1 -> Scope/2, Multiport Switch/2  "integrator t0"
  Integrator t1/1 -> Scope/3, Multiport Switch/3  "integrator t1"
  Integrator t2/1 -> Scope/4, Multiport Switch/4  "integrator t2"
  MATLAB Function1/2(x_dot1) -> Integrator t1/1
  MATLAB Function1/3(x_dot2) -> Integrator t2/1
  MATLAB Function/1(qNext) -> q/1  "q_before"
  q/1 -> MATLAB Function/1(q), Scope/5, Multiport Switch/1  "q_after"
  control/1 -> Scope/8, MATLAB Function/2(control)
  MATLAB Function/2(reset) -> reset/1
  reset/1 -> Integrator t0/2, Integrator t1/2, Integrator t2/2  "reset_after"

== system nuclearReactor/Plant28 ==
  control : Inport
  Integrator t0 : DiscreteIntegrator  ExternalReset=either  InitialConditionSource=external  InitialCondition=510  InitialConditionSetting=State (most efficient)  SampleTime=-1
  Integrator t1 : DiscreteIntegrator  ExternalReset=either  InitialConditionSource=external  InitialCondition=510  InitialConditionSetting=State (most efficient)  SampleTime=-1
  Integrator t2 : DiscreteIntegrator  ExternalReset=either  InitialConditionSource=external  InitialCondition=510  InitialConditionSetting=State (most efficient)  SampleTime=-1
  MATLAB Function : MATLAB Function  Priority=1  TreatAsAtomicUnit=on
  MATLAB Function1 : MATLAB Function  Priority=1  TreatAsAtomicUnit=on
  Multiport Switch : MultiPortSwitch  DataPortOrder=Zero-based contiguous
  Scope : Scope  NumInputPorts=8
      settings: TickLabels=on  ShowLegends=on  YMin=0~0~0~10~1~1~0~-1  YMax=40~20~20~30~3~3~1~1
  THR3 : Constant  Value=510
  THR4 : Constant  Value=550
  THR5 : Constant  Value=550
  q : Memory  LinearizeMemory=on
  reset : Memory  LinearizeMemory=on
  x : Outport
  wires:
  Multiport Switch/1 -> Scope/1, MATLAB Function1/1(x), x/1  "x"
  MATLAB Function1/1(x_dot0) -> Integrator t0/1
  THR3/1 -> Integrator t0/3
  THR4/1 -> Integrator t1/3
  THR5/1 -> Integrator t2/3
  Integrator t0/1 -> Scope/2, Multiport Switch/2  "integrator t0"
  Integrator t1/1 -> Scope/3, Multiport Switch/3  "integrator t1"
  Integrator t2/1 -> Scope/4, Multiport Switch/4  "integrator t2"
  MATLAB Function1/2(x_dot1) -> Integrator t1/1
  MATLAB Function1/3(x_dot2) -> Integrator t2/1
  MATLAB Function/1(qNext) -> q/1  "q_before"
  q/1 -> MATLAB Function/1(q), Scope/5, Multiport Switch/1  "q_after"
  control/1 -> Scope/8, MATLAB Function/2(control)
  MATLAB Function/2(reset) -> reset/1
  reset/1 -> Integrator t0/2, Integrator t1/2, Integrator t2/2  "reset_after"

== system nuclearReactor/Plant29 ==
  control : Inport
  Integrator t0 : DiscreteIntegrator  ExternalReset=either  InitialConditionSource=external  InitialCondition=510  InitialConditionSetting=State (most efficient)  SampleTime=-1
  Integrator t1 : DiscreteIntegrator  ExternalReset=either  InitialConditionSource=external  InitialCondition=510  InitialConditionSetting=State (most efficient)  SampleTime=-1
  Integrator t2 : DiscreteIntegrator  ExternalReset=either  InitialConditionSource=external  InitialCondition=510  InitialConditionSetting=State (most efficient)  SampleTime=-1
  MATLAB Function : MATLAB Function  Priority=1  TreatAsAtomicUnit=on
  MATLAB Function1 : MATLAB Function  Priority=1  TreatAsAtomicUnit=on
  Multiport Switch : MultiPortSwitch  DataPortOrder=Zero-based contiguous
  Scope : Scope  NumInputPorts=8
      settings: TickLabels=on  ShowLegends=on  YMin=0~0~0~10~1~1~0~-1  YMax=40~20~20~30~3~3~1~1
  THR3 : Constant  Value=510
  THR4 : Constant  Value=550
  THR5 : Constant  Value=550
  q : Memory  LinearizeMemory=on
  reset : Memory  LinearizeMemory=on
  x : Outport
  wires:
  Multiport Switch/1 -> Scope/1, MATLAB Function1/1(x), x/1  "x"
  MATLAB Function1/1(x_dot0) -> Integrator t0/1
  THR3/1 -> Integrator t0/3
  THR4/1 -> Integrator t1/3
  THR5/1 -> Integrator t2/3
  Integrator t0/1 -> Scope/2, Multiport Switch/2  "integrator t0"
  Integrator t1/1 -> Scope/3, Multiport Switch/3  "integrator t1"
  Integrator t2/1 -> Scope/4, Multiport Switch/4  "integrator t2"
  MATLAB Function1/2(x_dot1) -> Integrator t1/1
  MATLAB Function1/3(x_dot2) -> Integrator t2/1
  MATLAB Function/1(qNext) -> q/1  "q_before"
  q/1 -> MATLAB Function/1(q), Scope/5, Multiport Switch/1  "q_after"
  control/1 -> Scope/8, MATLAB Function/2(control)
  MATLAB Function/2(reset) -> reset/1
  reset/1 -> Integrator t0/2, Integrator t1/2, Integrator t2/2  "reset_after"

== system nuclearReactor/Plant3 ==
  control : Inport
  Integrator t0 : DiscreteIntegrator  ExternalReset=either  InitialConditionSource=external  InitialCondition=510  InitialConditionSetting=State (most efficient)  SampleTime=-1
  Integrator t1 : DiscreteIntegrator  ExternalReset=either  InitialConditionSource=external  InitialCondition=510  InitialConditionSetting=State (most efficient)  SampleTime=-1
  Integrator t2 : DiscreteIntegrator  ExternalReset=either  InitialConditionSource=external  InitialCondition=510  InitialConditionSetting=State (most efficient)  SampleTime=-1
  MATLAB Function : MATLAB Function  Priority=1  TreatAsAtomicUnit=on
  MATLAB Function1 : MATLAB Function  Priority=1  TreatAsAtomicUnit=on
  Multiport Switch : MultiPortSwitch  DataPortOrder=Zero-based contiguous
  Scope : Scope  NumInputPorts=8
      settings: TickLabels=on  ShowLegends=on  YMin=0~0~0~10~1~1~0~-1  YMax=40~20~20~30~3~3~1~1
  THR3 : Constant  Value=510
  THR4 : Constant  Value=550
  THR5 : Constant  Value=550
  q : Memory  LinearizeMemory=on
  reset : Memory  LinearizeMemory=on
  x : Outport
  wires:
  Multiport Switch/1 -> Scope/1, MATLAB Function1/1(x), x/1  "x"
  MATLAB Function1/1(x_dot0) -> Integrator t0/1
  THR3/1 -> Integrator t0/3
  THR4/1 -> Integrator t1/3
  THR5/1 -> Integrator t2/3
  Integrator t0/1 -> Scope/2, Multiport Switch/2  "integrator t0"
  Integrator t1/1 -> Scope/3, Multiport Switch/3  "integrator t1"
  Integrator t2/1 -> Scope/4, Multiport Switch/4  "integrator t2"
  MATLAB Function1/2(x_dot1) -> Integrator t1/1
  MATLAB Function1/3(x_dot2) -> Integrator t2/1
  MATLAB Function/1(qNext) -> q/1  "q_before"
  q/1 -> MATLAB Function/1(q), Scope/5, Multiport Switch/1  "q_after"
  control/1 -> Scope/8, MATLAB Function/2(control)
  MATLAB Function/2(reset) -> reset/1
  reset/1 -> Integrator t0/2, Integrator t1/2, Integrator t2/2  "reset_after"

== system nuclearReactor/Plant4 ==
  control : Inport
  Integrator t0 : DiscreteIntegrator  ExternalReset=either  InitialConditionSource=external  InitialCondition=510  InitialConditionSetting=State (most efficient)  SampleTime=-1
  Integrator t1 : DiscreteIntegrator  ExternalReset=either  InitialConditionSource=external  InitialCondition=510  InitialConditionSetting=State (most efficient)  SampleTime=-1
  Integrator t2 : DiscreteIntegrator  ExternalReset=either  InitialConditionSource=external  InitialCondition=510  InitialConditionSetting=State (most efficient)  SampleTime=-1
  MATLAB Function : MATLAB Function  Priority=1  TreatAsAtomicUnit=on
  MATLAB Function1 : MATLAB Function  Priority=1  TreatAsAtomicUnit=on
  Multiport Switch : MultiPortSwitch  DataPortOrder=Zero-based contiguous
  Scope : Scope  NumInputPorts=8
      settings: TickLabels=on  ShowLegends=on  YMin=0~0~0~10~1~1~0~-1  YMax=40~20~20~30~3~3~1~1
  THR3 : Constant  Value=510
  THR4 : Constant  Value=550
  THR5 : Constant  Value=550
  q : Memory  LinearizeMemory=on
  reset : Memory  LinearizeMemory=on
  x : Outport
  wires:
  Multiport Switch/1 -> Scope/1, MATLAB Function1/1(x), x/1  "x"
  MATLAB Function1/1(x_dot0) -> Integrator t0/1
  THR3/1 -> Integrator t0/3
  THR4/1 -> Integrator t1/3
  THR5/1 -> Integrator t2/3
  Integrator t0/1 -> Scope/2, Multiport Switch/2  "integrator t0"
  Integrator t1/1 -> Scope/3, Multiport Switch/3  "integrator t1"
  Integrator t2/1 -> Scope/4, Multiport Switch/4  "integrator t2"
  MATLAB Function1/2(x_dot1) -> Integrator t1/1
  MATLAB Function1/3(x_dot2) -> Integrator t2/1
  MATLAB Function/1(qNext) -> q/1  "q_before"
  q/1 -> MATLAB Function/1(q), Scope/5, Multiport Switch/1  "q_after"
  control/1 -> Scope/8, MATLAB Function/2(control)
  MATLAB Function/2(reset) -> reset/1
  reset/1 -> Integrator t0/2, Integrator t1/2, Integrator t2/2  "reset_after"

== system nuclearReactor/Plant5 ==
  control : Inport
  Integrator t0 : DiscreteIntegrator  ExternalReset=either  InitialConditionSource=external  InitialCondition=510  InitialConditionSetting=State (most efficient)  SampleTime=-1
  Integrator t1 : DiscreteIntegrator  ExternalReset=either  InitialConditionSource=external  InitialCondition=510  InitialConditionSetting=State (most efficient)  SampleTime=-1
  Integrator t2 : DiscreteIntegrator  ExternalReset=either  InitialConditionSource=external  InitialCondition=510  InitialConditionSetting=State (most efficient)  SampleTime=-1
  MATLAB Function : MATLAB Function  Priority=1  TreatAsAtomicUnit=on
  MATLAB Function1 : MATLAB Function  Priority=1  TreatAsAtomicUnit=on
  Multiport Switch : MultiPortSwitch  DataPortOrder=Zero-based contiguous
  Scope : Scope  NumInputPorts=8
      settings: TickLabels=on  ShowLegends=on  YMin=0~0~0~10~1~1~0~-1  YMax=40~20~20~30~3~3~1~1
  THR3 : Constant  Value=510
  THR4 : Constant  Value=550
  THR5 : Constant  Value=550
  q : Memory  LinearizeMemory=on
  reset : Memory  LinearizeMemory=on
  x : Outport
  wires:
  Multiport Switch/1 -> Scope/1, MATLAB Function1/1(x), x/1  "x"
  MATLAB Function1/1(x_dot0) -> Integrator t0/1
  THR3/1 -> Integrator t0/3
  THR4/1 -> Integrator t1/3
  THR5/1 -> Integrator t2/3
  Integrator t0/1 -> Scope/2, Multiport Switch/2  "integrator t0"
  Integrator t1/1 -> Scope/3, Multiport Switch/3  "integrator t1"
  Integrator t2/1 -> Scope/4, Multiport Switch/4  "integrator t2"
  MATLAB Function1/2(x_dot1) -> Integrator t1/1
  MATLAB Function1/3(x_dot2) -> Integrator t2/1
  MATLAB Function/1(qNext) -> q/1  "q_before"
  q/1 -> MATLAB Function/1(q), Scope/5, Multiport Switch/1  "q_after"
  control/1 -> Scope/8, MATLAB Function/2(control)
  MATLAB Function/2(reset) -> reset/1
  reset/1 -> Integrator t0/2, Integrator t1/2, Integrator t2/2  "reset_after"
